simulink model "amesimcar_pathplanner_constspeed_MPC"  (R2018a)
settings: Solver=VariableStepAuto  StartTime=0.0  StopTime=300  RelTol=1e-3
values from neighbouring files (symbols this model uses):
  ref_vel = zeros(1,100)    [Planning2.m]    (also in Planning3_constspeed.m)
undefined symbols (not defined in the file or in its folder): centerline1, centerline2, left_line, middle_line, phi0, right_line, v0, x0, y0
settings Model: Creator=pm6kgn  LastModifiedBy=pm6kgn

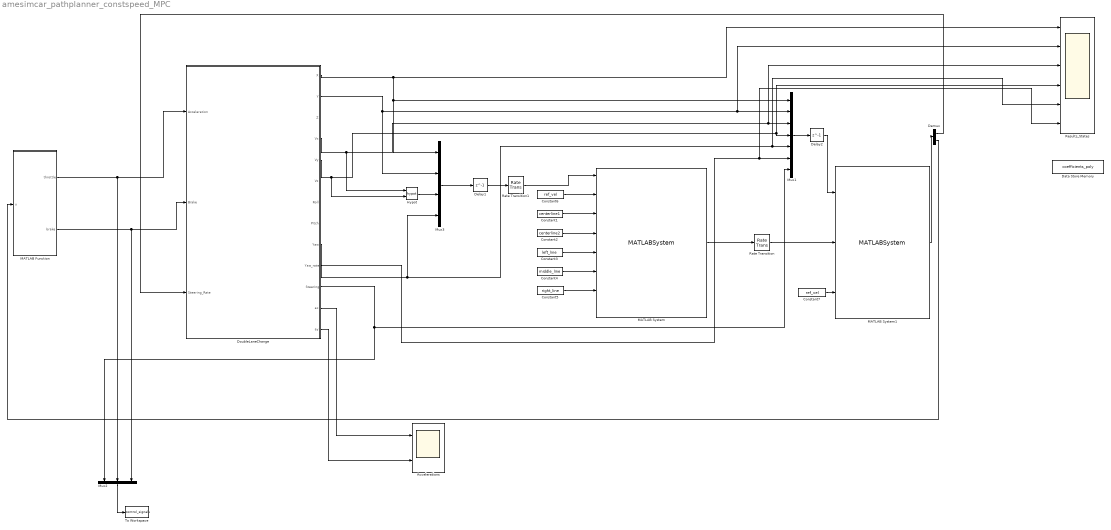
== system amesimcar_pathplanner_constspeed_MPC ==
  Accelerations : Scope  NumInputPorts=2
  Constant1 : Constant  Value=centerline1
  Constant2 : Constant  Value=centerline2
  Constant3 : Constant  Value=left_line
  Constant4 : Constant  Value=middle_line
  Constant5 : Constant  Value=right_line
  Constant6 : Constant  Value=ref_vel
  Constant7 : Constant  Value=ref_vel
  Data Store Memory : DataStoreMemory  DataStoreName=coefficients_poly  ReadBeforeWriteMsg=warning  WriteAfterWriteMsg=warning  WriteAfterReadMsg=warning  InitialValue=zeros(8,1)  ShareAcrossModelInstances=on  ShowAdditionalParam=off  OutDataTypeStr=double
  Delay1 : Delay  DelayLength=1  InitialCondition=[x0;y0;v0;phi0]
  Delay2 : Delay  DelayLength=1  InitialCondition=[x0;y0;v0;0;phi0;0;0]
  Demux : Demux  Outputs=2
  DoubleLaneChange : Subsystem  Tag=AME2SLCoSim  InitFcn=AMESimLib_initBlock  StartFcn=AMESimLib_startBlock  StopFcn=AMESimLib_stopBlock
      settings: DeleteFcn=AMESimLib_deleteBlock  OpenFcn=AMESimLib_openBlock('AME2SLCoSim')
      mask Display: image(imread('amesim_pix256.png'),[0.4,0.7,0.2,0.2]);disp('Simcenter Amesim co-Sim:\nDoubleLaneChange');port_label('input',1,'Acceleration');port_label('input',2,'Brake');port_label('input',3,'Steering_Rate');port_label('output',1,'X');port_label('output',2,'Y');port_label('output',3,'Z');port_label('output',4,'Vx');port_label('output',5,'Vy');port_label('output',6,'Vz');port_label('output',7,'Roll');port_label('output',8,'Pitch');port_label('output',9,'Yaw');port_label('output',10,'Yaw_rate');port_label('output',11,'Steering');port_label('output',12,'ax');port_label('output',13,'ay');
  Hypot : Math  Operator=hypot  SaturateOnIntegerOverflow=on
  MATLAB Function : MATLAB Function  TreatAsAtomicUnit=on
  MATLAB System : MATLABSystem  System=Planning2_working_constspeed  SimulateUsing=Interpreted execution
      mask Type: Planning2_working_constspeed
      mask Display:
      | disp('Planning2_working_constspeed');
      | port_label('input',1,'current_states');
      | port_label('input',2,'reference_velocity');
      | port_label('input',3,'centerline1');
      | port_label('input',4,'centerline2');
      | port_label('input',5,'left_line');
      | port_label('input',6,'middle_line');
      | port_label('input',7,'right_line');
      | port_label('input',8,'time');
      | port_label('output',1,'reference');
  MATLAB System1 : MATLABSystem  System=Tracker_working_constspeed  SimulateUsing=Interpreted execution
      mask Type: Tracker_working_constspeed
      mask Display:
      | disp('Tracker_working_constspeed');
      | port_label('input',1,'current_states');
      | port_label('input',2,'reference');
      | port_label('input',3,'ref_vel');
      | port_label('output',1,'control');
  Mux1 : Mux  Inputs=7
  Mux2 : Mux  Inputs=3
  Mux3 : Mux
  Rate Transition : RateTransition
  Rate Transition1 : RateTransition
  Results_States : Scope  NumInputPorts=6
  To Workspace : ToWorkspace  VariableName=control_signals  SaveFormat=Structure With Time  SampleTime=-1
  wires:
  DoubleLaneChange/4(Vx) -> Hypot/1, Results_States/3, Mux1/3
  DoubleLaneChange/9(Yaw) -> Mux3/4, Mux1/5, Results_States/5
  DoubleLaneChange/1(X) -> Mux3/1, Mux1/1, Results_States/1
  Delay1/1 -> Rate Transition1/1
  Demux/2 -> MATLAB Function/1(u)
  DoubleLaneChange/12(ax) -> Accelerations/1
  Constant5/1 -> MATLAB System/7
  Constant3/1 -> MATLAB System/5
  DoubleLaneChange/13(ay) -> Accelerations/2
  Mux3/1 -> Delay1/1
  DoubleLaneChange/2(Y) -> Mux3/2, Results_States/2, Mux1/2
  Rate Transition1/1 -> MATLAB System/1
  DoubleLaneChange/11(Steering) -> Mux1/7, Mux2/1
  MATLAB Function/1(throttle) -> Mux2/2, DoubleLaneChange/1(Acceleration)
  Constant7/1 -> MATLAB System1/3
  Delay2/1 -> MATLAB System1/1
  MATLAB System/1 -> Rate Transition/1
  DoubleLaneChange/10(Yaw_rate) -> Results_States/6, Mux1/6
  Constant4/1 -> MATLAB System/6
  Constant1/1 -> MATLAB System/3
  Hypot/1 -> Mux3/3
  Constant2/1 -> MATLAB System/4
  MATLAB Function/2(brake) -> Mux2/3, DoubleLaneChange/2(Brake)
  Rate Transition/1 -> MATLAB System1/2
  Mux2/1 -> To Workspace/1
  Mux1/1 -> Delay2/1
  Demux/1 -> DoubleLaneChange/3(Steering_Rate)
  DoubleLaneChange/5(Vy) -> Mux1/4, Results_States/4, Hypot/2
  MATLAB System1/1 -> Demux/1
  Constant6/1 -> MATLAB System/2

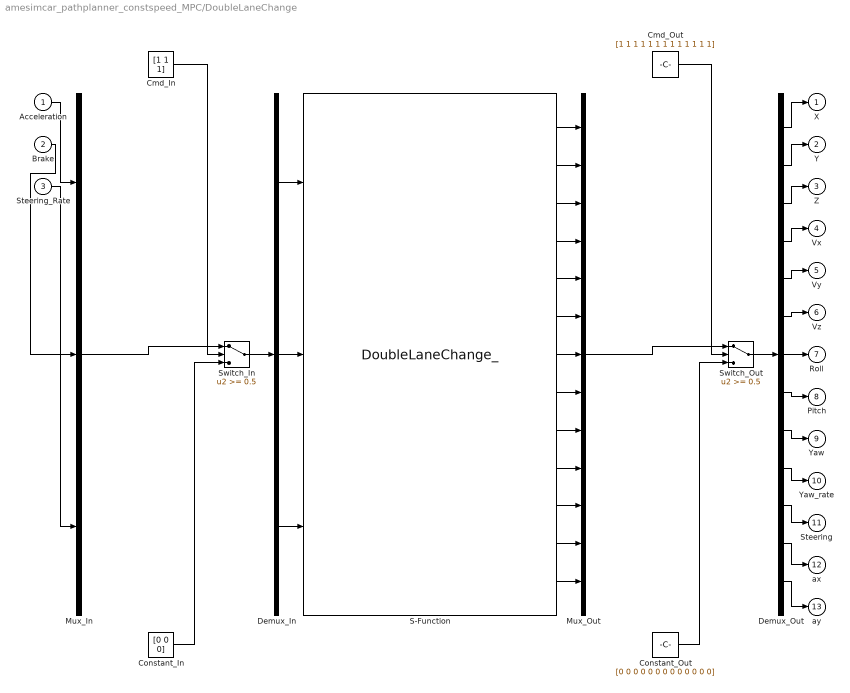
== system amesimcar_pathplanner_constspeed_MPC/DoubleLaneChange ==
  Acceleration : Inport
  Brake : Inport  Port=2
  Steering_Rate : Inport  Port=3
  Cmd_In : Constant  Value=[1 1 1]
  Cmd_Out : Constant  Value=[1 1 1 1 1 1 1 1 1 1 1 1 1]
  Constant_In : Constant  Value=[0 0 0]
  Constant_Out : Constant  Value=[0 0 0 0 0 0 0 0 0 0 0 0 0]
  Demux_In : Demux  Outputs=3
  Demux_Out : Demux  Outputs=13
  Mux_In : Mux  Inputs=3
  Mux_Out : Mux  Inputs=13
  S-Function : S-Function  InitFcn=clear DoubleLaneChange_  StopFcn=clear DoubleLaneChange_  FunctionName=DoubleLaneChange_  Parameters="[0.01;0.01;1e-05;1e+30;100;0;0;2;0;1;0.001;0;1] ['Grav           ';'Xg             ';'Zg             ';'Msprung        ';'Msteer         ';'Msp_front      ';'Mwh_front      ';'Msp_rear       ';'Mwh_rear       ';'Isprung_xx     ';'Isprung_yy     ';'Isprung_zz     ';'Isprung_xy     ';'Isprung_xz     ';'Isprung_yz     ';'Zref_front     ';'Zref_rear      ';'wheelbase      ';'track_front    ';'track_rear     ';'Rpinion        ';'Ksusp_front    ';'Ksusp_rear     ';'Rsusp_front    ';'Rsusp_rear     ';'Kantiroll_front';'Kantiroll_rear ';'Rfree          ';'Rroll          ';'Ktire          ';'Rtire          ';'a1             ';'a2             ';'a3             ';'a4             '] [9.8066;1056;375;1300;2;18;18;15;14;250;1000;1300;0;-20;0;75;75;2400;1450;1450;8;21000;21000;2000;1500;30000;20000;0.292;0.291;200000;100;-50;1200;1000;5] [] [] [] []"  SFunctionDeploymentMode=off  EnableBusSupport=off
      mask Display: port_label('output',1,'X');port_label('output',2,'Y');port_label('output',3,'Z');port_label('output',4,'Vx');port_label('output',5,'Vy');port_label('output',6,'Vz');port_label('output',7,'Roll');port_label('output',8,'Pitch');port_label('output',9,'Yaw');port_label('output',10,'Yaw_rate');port_label('output',11,'Steering');port_label('output',12,'ax');port_label('output',13,'ay');port_label('input',1,'Acceleration');port_label('input',2,'Brake');port_label('input',3,'Steering_Rate');disp('Simcenter Amesim:\n DoubleLaneChange_')
  Switch_In : Switch  Threshold=0.5  SaturateOnIntegerOverflow=on  InputSameDT=on
  Switch_Out : Switch  Threshold=0.5  SaturateOnIntegerOverflow=on  InputSameDT=on
  X : Outport
  Y : Outport  Port=2
  Z : Outport  Port=3
  Vx : Outport  Port=4
  Vy : Outport  Port=5
  Vz : Outport  Port=6
  Roll : Outport  Port=7
  Pitch : Outport  Port=8
  Yaw : Outport  Port=9
  Yaw_rate : Outport  Port=10
  Steering : Outport  Port=11
  ax : Outport  Port=12
  ay : Outport  Port=13
  wires:
  Mux_In/1 -> Switch_In/1
  Cmd_In/1 -> Switch_In/2
  Constant_In/1 -> Switch_In/3
  Switch_In/1 -> Demux_In/1
  Mux_Out/1 -> Switch_Out/1
  Cmd_Out/1 -> Switch_Out/2
  Constant_Out/1 -> Switch_Out/3
  Switch_Out/1 -> Demux_Out/1
  Acceleration/1 -> Mux_In/1
  Demux_In/1 -> S-Function/1
  Brake/1 -> Mux_In/2
  Demux_In/2 -> S-Function/2
  Steering_Rate/1 -> Mux_In/3
  Demux_In/3 -> S-Function/3
  Demux_Out/1 -> X/1
  S-Function/1 -> Mux_Out/1
  Demux_Out/2 -> Y/1
  S-Function/2 -> Mux_Out/2
  Demux_Out/3 -> Z/1
  S-Function/3 -> Mux_Out/3
  Demux_Out/4 -> Vx/1
  S-Function/4 -> Mux_Out/4
  Demux_Out/5 -> Vy/1
  S-Function/5 -> Mux_Out/5
  Demux_Out/6 -> Vz/1
  S-Function/6 -> Mux_Out/6
  Demux_Out/7 -> Roll/1
  S-Function/7 -> Mux_Out/7
  Demux_Out/8 -> Pitch/1
  S-Function/8 -> Mux_Out/8
  Demux_Out/9 -> Yaw/1
  S-Function/9 -> Mux_Out/9
  Demux_Out/10 -> Yaw_rate/1
  S-Function/10 -> Mux_Out/10
  Demux_Out/11 -> Steering/1
  S-Function/11 -> Mux_Out/11
  Demux_Out/12 -> ax/1
  S-Function/12 -> Mux_Out/12
  Demux_Out/13 -> ay/1
  S-Function/13 -> Mux_Out/13

== matlab function amesimcar_pathplanner_constspeed_MPC/MATLAB Function ==
  data: u input; throttle output; brake output
function [throttle, brake]= fcn(u)
%#codegen

if u >= 0
    throttle = u;
    brake = 0;
else
    brake = -u;
    throttle = 0;
end

end
